simulink model "testharness"  (R2023a)
settings: Solver=ode4  StartTime=0.0  StopTime=30  FixedStep=sim.sample_time_s  RelTol=1e-3
undefined symbols (not defined in the file): rot_K_meas_IB_B_radDs, sfor_meas_B_mDs2, sim
libraries: simulink x5, lib_kinematics x2, matrix_library x1
settings Model: PauseTimes=16  Creator=FC_dev1  LastModifiedBy=FC_dev1

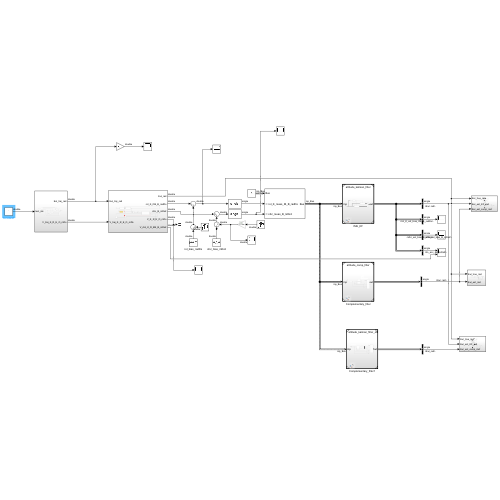
[thumbnail: Simulink's stored preview of the top-level diagram]
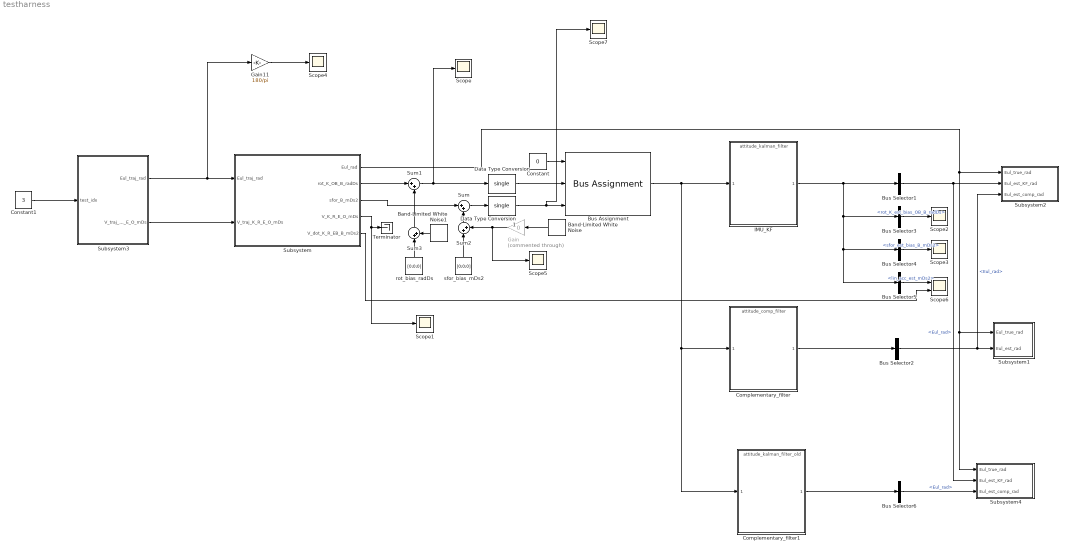
== system testharness ==
  Band-Limited White Noise : simulink/Sources/Band-Limited White Noise  Cov=meas_acc_var  Ts=0.1  seed=[1 2 3]
  Band-Limited White Noise1 : simulink/Sources/Band-Limited White Noise  Cov=rot_var  Ts=0.1  seed=[1 2 3]
  Bus Assignment : BusAssignment  AssignedSignals=rot_K_meas_IB_B_radDs,sfor_meas_B_mDs2
  Bus Selector1 : BusSelector  OutputSignals=Eul_rad
  Bus Selector2 : BusSelector  OutputSignals=Eul_rad
  Bus Selector3 : BusSelector  OutputSignals=rot_K_est_bias_OB_B_radDs
  Bus Selector4 : BusSelector  OutputSignals=sfor_est_bias_B_mDs2
  Bus Selector5 : BusSelector  OutputSignals=lin_acc_est_mDs2
  Bus Selector6 : BusSelector  OutputSignals=Eul_rad
  Complementary_filter : ModelReference  ModelNameDialog=attitude_comp_filter.slx  SimulationMode=Normal  ModelReferenceVersion=1.222
  Complementary_filter1 : ModelReference  ModelNameDialog=attitude_kalman_filter_old.slx  SimulationMode=Normal  ModelReferenceVersion=1.208
  Constant : Constant  Value=0  OutDataTypeStr=Bus: inp_Bus
  Constant1 : Constant  Value=3
  Data Type Conversion : DataTypeConversion  OutDataTypeStr=single  SaturateOnIntegerOverflow=off  RndMeth=Floor
  Data Type Conversion1 : DataTypeConversion  OutDataTypeStr=single  SaturateOnIntegerOverflow=off  RndMeth=Floor
  Gain : Gain  Commented=through  Gain=0
  Gain11 : Gain  Gain=180/pi
  IMU_KF : ModelReference  ModelNameDialog=attitude_kalman_filter.slx  SimulationMode=Normal  ModelReferenceVersion=1.336
  Scope{,1..5,7} (7 alike) : Scope
  Scope6 : Scope  NumInputPorts=2
  Subsystem : Subsystem
  Subsystem1 : Subsystem
  Subsystem2 : Subsystem
  Subsystem3 : Subsystem
  Subsystem4 : Subsystem
  Sum{,1..3} (4 alike) : Sum  Inputs=|++
  Terminator : Terminator
  rot_bias_radDs : Constant  Value=[0;0;0]  VectorParams1D=off
  sfor_bias_mDs2 : Constant  Value=[0;0;0]  VectorParams1D=off
  wires:
  Constant/1 -> Bus Assignment/1
  Bus Assignment/1 -> Complementary_filter1/1, Complementary_filter/1, IMU_KF/1
  Data Type Conversion/1 -> Bus Assignment/2
  Data Type Conversion1/1 -> Scope7/1, Bus Assignment/3
  Subsystem/1(Eul_rad) -> Subsystem4/1(Eul_true_rad), Subsystem1/1(Eul_true_rad), Subsystem2/1(Eul_true_rad)
  Subsystem/2(rot_K_OB_B_radDs) -> Sum1/1
  Subsystem/3(sfor_B_mDs2) -> Sum/1
  IMU_KF/1 -> Bus Selector3/1, Bus Selector5/1, Bus Selector4/1, Bus Selector1/1
  Bus Selector1/1 -> Subsystem4/2(Eul_est_KF_rad), Subsystem2/2(Eul_est_KF_rad)  "<Eul_rad>"
  Bus Selector3/1 -> Scope2/1  "<rot_K_est_bias_OB_B_radDs>"
  Bus Selector4/1 -> Scope3/1  "<sfor_est_bias_B_mDs2>"
  Gain11/1 -> Scope4/1
  Subsystem/4(V_K_R_E_O_mDs) -> Scope1/1, Terminator/1
  Sum/1 -> Data Type Conversion1/1
  Sum1/1 -> Data Type Conversion/1, Scope/1
  rot_bias_radDs/1 -> Sum3/1
  sfor_bias_mDs2/1 -> Sum2/1
  Complementary_filter/1 -> Bus Selector2/1
  Bus Selector2/1 -> Subsystem2/3(Eul_est_comp_rad), Subsystem1/2(Eul_est_rad)  "<Eul_rad>"
  Subsystem3/1(Eul_traj_rad) -> Gain11/1, Subsystem/1(Eul_traj_rad)
  Subsystem3/2(V_traj_K_R_E_O_mDs) -> Subsystem/2(V_traj_K_R_E_O_mDs)
  Constant1/1 -> Subsystem3/1(test_idx)
  Sum2/1 -> Sum/2
  Band-Limited White Noise/1 -> Gain/1
  Sum3/1 -> Sum1/2
  Band-Limited White Noise1/1 -> Sum3/2
  Complementary_filter1/1 -> Bus Selector6/1
  Bus Selector6/1 -> Subsystem4/3(Eul_est_comp_rad)  "<Eul_rad>"
  Bus Selector5/1 -> Scope6/1  "<lin_acc_est_mDs2>"
  Subsystem/5(V_dot_K_R_EB_B_mDs2) -> Scope6/2
  Gain/1 -> Scope5/1, Sum2/2

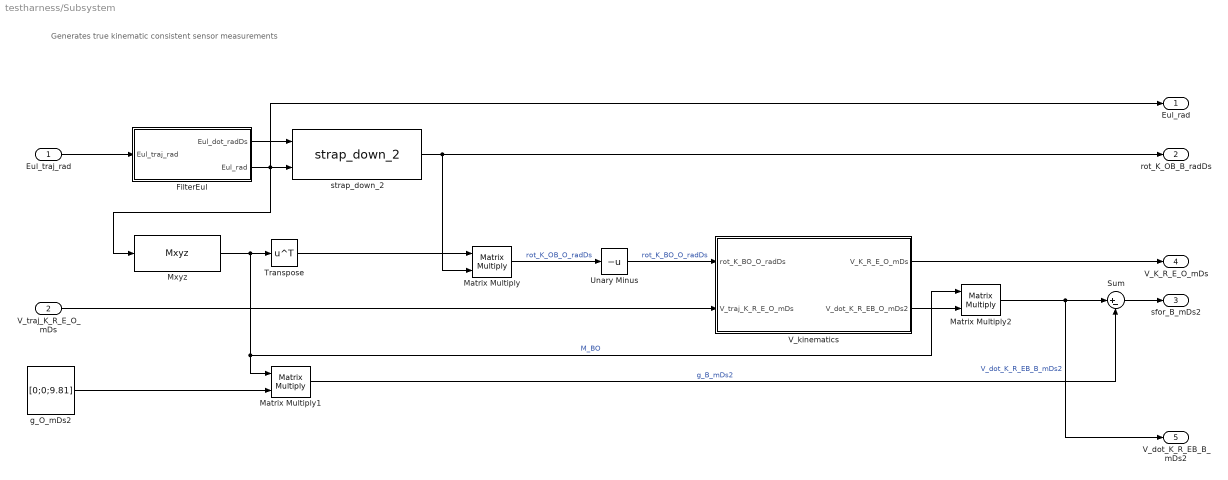
== system testharness/Subsystem ==
  note: Generates true kinematic consistent sensor measurements
  Eul_traj_rad : Inport
  V_traj_K_R_E_O_mDs : Inport  Port=2
  FilterEul : Subsystem
  Matrix Multiply : Product  Multiplication=Matrix(*)
  Matrix Multiply1 : Product  Multiplication=Matrix(*)
  Matrix Multiply2 : Product  Multiplication=Matrix(*)
  Mxyz : lib_kinematics/Mxyz  SystemSampleTime=-1  VariantActivationTime=update diagram  Latency=0  AutoFrameSizeCalculation=off
  Sum : Sum  Inputs=|+-
  Transpose : Math  Operator=transpose
  Unary Minus : UnaryMinus
  V_kinematics : Subsystem
  g_O_mDs2 : Constant  Value=[0;0;9.81]  VectorParams1D=off
  strap_down_2 : lib_kinematics/strap_down_2  SystemSampleTime=-1  VariantActivationTime=update diagram  Latency=0  AutoFrameSizeCalculation=off
  Eul_rad : Outport
  rot_K_OB_B_radDs : Outport  Port=2
  sfor_B_mDs2 : Outport  Port=3
  V_K_R_E_O_mDs : Outport  Port=4
  V_dot_K_R_EB_B_mDs2 : Outport  Port=5
  wires:
  Eul_traj_rad/1 -> FilterEul/1(Eul_traj_rad)
  V_traj_K_R_E_O_mDs/1 -> V_kinematics/2(V_traj_K_R_E_O_mDs)
  FilterEul/1(Eul_dot_radDs) -> strap_down_2/1
  FilterEul/2(Eul_rad) -> Mxyz/1, Eul_rad/1, strap_down_2/2
  Mxyz/1 -> Matrix Multiply2/1, Matrix Multiply1/1, Transpose/1  "M_BO"
  Transpose/1 -> Matrix Multiply/1
  strap_down_2/1 -> rot_K_OB_B_radDs/1, Matrix Multiply/2
  Matrix Multiply/1 -> Unary Minus/1  "rot_K_OB_O_radDs"
  Unary Minus/1 -> V_kinematics/1(rot_K_BO_O_radDs)  "rot_K_BO_O_radDs"
  g_O_mDs2/1 -> Matrix Multiply1/2
  Matrix Multiply1/1 -> Sum/2  "g_B_mDs2"
  Sum/1 -> sfor_B_mDs2/1
  V_kinematics/2(V_dot_K_R_EB_O_mDs2) -> Matrix Multiply2/2
  Matrix Multiply2/1 -> V_dot_K_R_EB_B_mDs2/1, Sum/1  "V_dot_K_R_EB_B_mDs2"
  V_kinematics/1(V_K_R_E_O_mDs) -> V_K_R_E_O_mDs/1

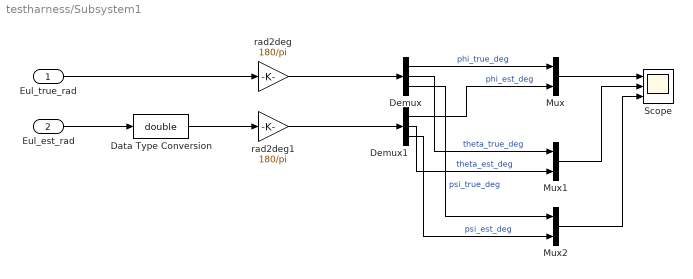
== system testharness/Subsystem1 ==
  Eul_true_rad : Inport
  Eul_est_rad : Inport  Port=2
  Data Type Conversion : DataTypeConversion  OutDataTypeStr=double  SaturateOnIntegerOverflow=off  RndMeth=Floor
  Demux : Demux  Outputs=3
  Demux1 : Demux  Outputs=3
  Mux : Mux  Inputs=2
  Mux1 : Mux  Inputs=2
  Mux2 : Mux  Inputs=2
  Scope : Scope  NumInputPorts=3
  rad2deg : Gain  Gain=180/pi  OutDataTypeStr=Inherit: Same as input
  rad2deg1 : Gain  Gain=180/pi  OutDataTypeStr=Inherit: Same as input
  wires:
  Eul_est_rad/1 -> Data Type Conversion/1
  Eul_true_rad/1 -> rad2deg/1
  rad2deg/1 -> Demux/1
  rad2deg1/1 -> Demux1/1
  Demux/1 -> Mux/1  "phi_true_deg"
  Demux1/1 -> Mux/2  "phi_est_deg"
  Demux/2 -> Mux1/1  "theta_true_deg"
  Demux1/2 -> Mux1/2  "theta_est_deg"
  Demux/3 -> Mux2/1  "psi_true_deg"
  Demux1/3 -> Mux2/2  "psi_est_deg"
  Mux/1 -> Scope/1
  Mux1/1 -> Scope/2
  Mux2/1 -> Scope/3
  Data Type Conversion/1 -> rad2deg1/1

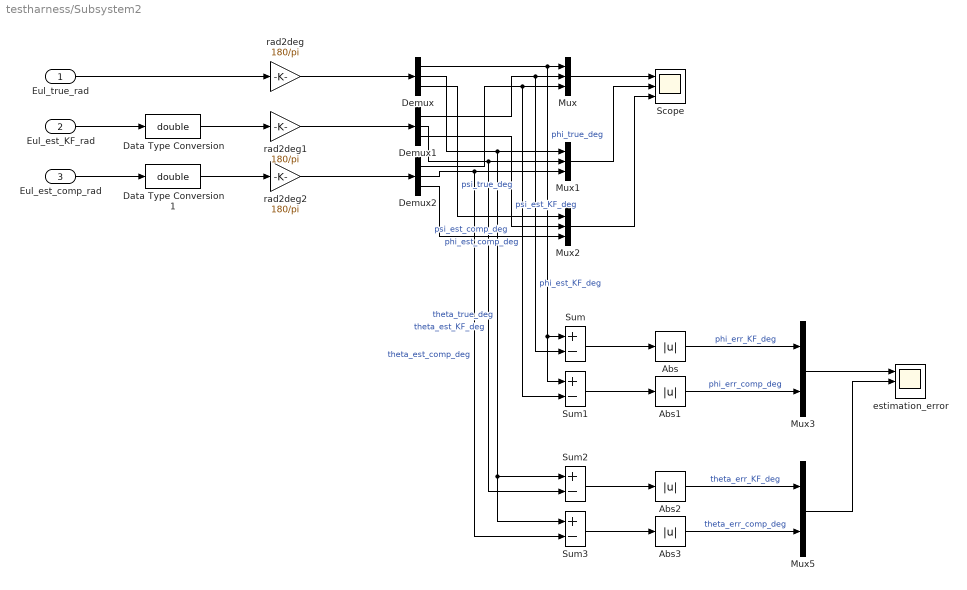
== system testharness/Subsystem2 ==
  Eul_true_rad : Inport
  Eul_est_KF_rad : Inport  Port=2
  Eul_est_comp_rad : Inport  Port=3
  Abs{,1..3} (4 alike) : Abs  SaturateOnIntegerOverflow=off
  Data Type Conversion : DataTypeConversion  OutDataTypeStr=double  SaturateOnIntegerOverflow=off  RndMeth=Floor
  Data Type Conversion1 : DataTypeConversion  OutDataTypeStr=double  SaturateOnIntegerOverflow=off  RndMeth=Floor
  Demux : Demux  Outputs=3
  Demux1 : Demux  Outputs=3
  Demux2 : Demux  Outputs=3
  Mux : Mux  Inputs=3
  Mux1 : Mux  Inputs=3
  Mux2 : Mux  Inputs=3
  Mux3 : Mux  Inputs=2
  Mux5 : Mux  Inputs=2
  Scope : Scope  NumInputPorts=3
  Sum{,1..3} (4 alike) : Sum  Inputs=+-
  estimation_error : Scope  NumInputPorts=3
  rad2deg : Gain  Gain=180/pi  OutDataTypeStr=Inherit: Same as input
  rad2deg1 : Gain  Gain=180/pi  OutDataTypeStr=Inherit: Same as input
  rad2deg2 : Gain  Gain=180/pi  OutDataTypeStr=Inherit: Same as input
  wires:
  Data Type Conversion/1 -> rad2deg1/1
  Mux2/1 -> Scope/3
  Mux1/1 -> Scope/2
  Mux/1 -> Scope/1
  Demux1/3 -> Mux2/2  "psi_est_KF_deg"
  Demux/3 -> Mux2/1  "psi_true_deg"
  Demux1/2 -> Sum2/2, Mux1/2  "theta_est_KF_deg"
  Demux/2 -> Sum3/1, Sum2/1, Mux1/1  "theta_true_deg"
  Demux1/1 -> Sum/2, Mux/2  "phi_est_KF_deg"
  Demux/1 -> Sum1/1, Sum/1, Mux/1  "phi_true_deg"
  rad2deg1/1 -> Demux1/1
  rad2deg/1 -> Demux/1
  Eul_true_rad/1 -> rad2deg/1
  Eul_est_KF_rad/1 -> Data Type Conversion/1
  Eul_est_comp_rad/1 -> Data Type Conversion1/1
  Data Type Conversion1/1 -> rad2deg2/1
  rad2deg2/1 -> Demux2/1
  Demux2/1 -> Sum1/2, Mux/3  "phi_est_comp_deg"
  Demux2/2 -> Mux1/3, Sum3/2  "theta_est_comp_deg"
  Demux2/3 -> Mux2/3  "psi_est_comp_deg"
  Sum/1 -> Abs/1
  Abs/1 -> Mux3/1  "phi_err_KF_deg"
  Sum1/1 -> Abs1/1
  Abs1/1 -> Mux3/2  "phi_err_comp_deg"
  Mux3/1 -> estimation_error/1
  Sum2/1 -> Abs2/1
  Sum3/1 -> Abs3/1
  Abs2/1 -> Mux5/1  "theta_err_KF_deg"
  Abs3/1 -> Mux5/2  "theta_err_comp_deg"
  Mux5/1 -> estimation_error/2

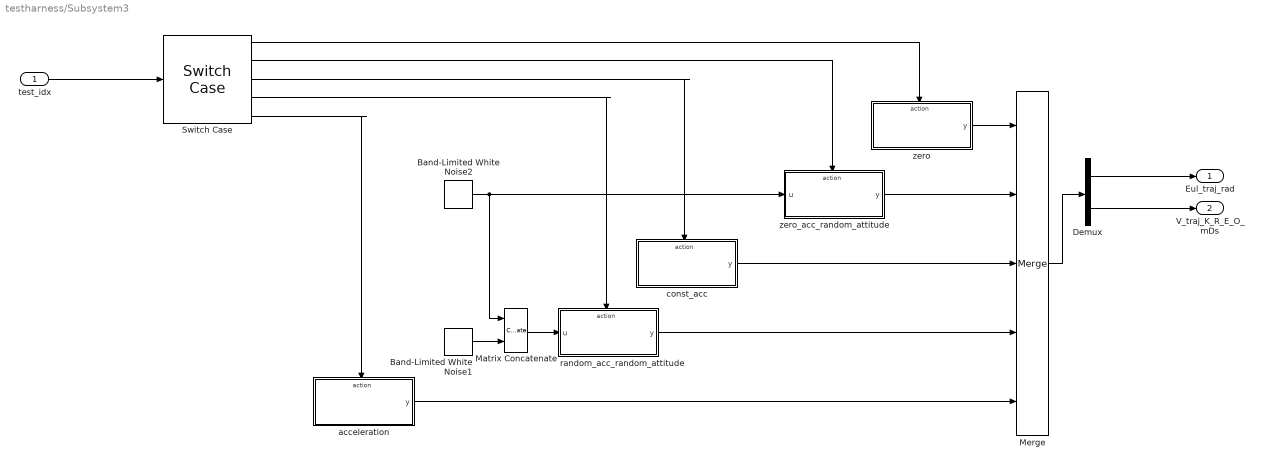
== system testharness/Subsystem3 ==
  test_idx : Inport
  Band-Limited White Noise1 : simulink/Sources/Band-Limited White Noise  Cov=[1 1 1]*5  Ts=sim.sample_time_s  seed=[23344 23345 23346]
  Band-Limited White Noise2 : simulink/Sources/Band-Limited White Noise  Cov=[0.01 0.01 0.01]  Ts=sim.sample_time_s  seed=[23341 23342 23343]
  Demux : Demux  Outputs=2
  Matrix Concatenate : Concatenate  Mode=Multidimensional array
  Merge : Merge  Inputs=5
  Switch Case : SwitchCase  CaseConditions={0,1,2,3,4}  ShowDefaultCase=off
  acceleration : Subsystem  TreatAsAtomicUnit=on
  const_acc : Subsystem  TreatAsAtomicUnit=on
  random_acc_random_attitude : Subsystem  TreatAsAtomicUnit=on
  zero : Subsystem  TreatAsAtomicUnit=on
  zero_acc_random_attitude : Subsystem  TreatAsAtomicUnit=on
  Eul_traj_rad : Outport
  V_traj_K_R_E_O_mDs : Outport  Port=2
  wires:
  test_idx/1 -> Switch Case/1
  Switch Case/3 -> const_acc/Action
  Switch Case/2 -> zero_acc_random_attitude/Action
  Switch Case/1 -> zero/Action
  zero/1(y) -> Merge/1
  zero_acc_random_attitude/1(y) -> Merge/2
  const_acc/1(y) -> Merge/3
  Merge/1 -> Demux/1
  Demux/1 -> Eul_traj_rad/1
  Demux/2 -> V_traj_K_R_E_O_mDs/1
  Band-Limited White Noise2/1 -> Matrix Concatenate/1, zero_acc_random_attitude/1(u)
  random_acc_random_attitude/1(y) -> Merge/4
  Switch Case/4 -> random_acc_random_attitude/Action
  Band-Limited White Noise1/1 -> Matrix Concatenate/2
  Matrix Concatenate/1 -> random_acc_random_attitude/1(u)
  acceleration/1(y) -> Merge/5
  Switch Case/5 -> acceleration/Action

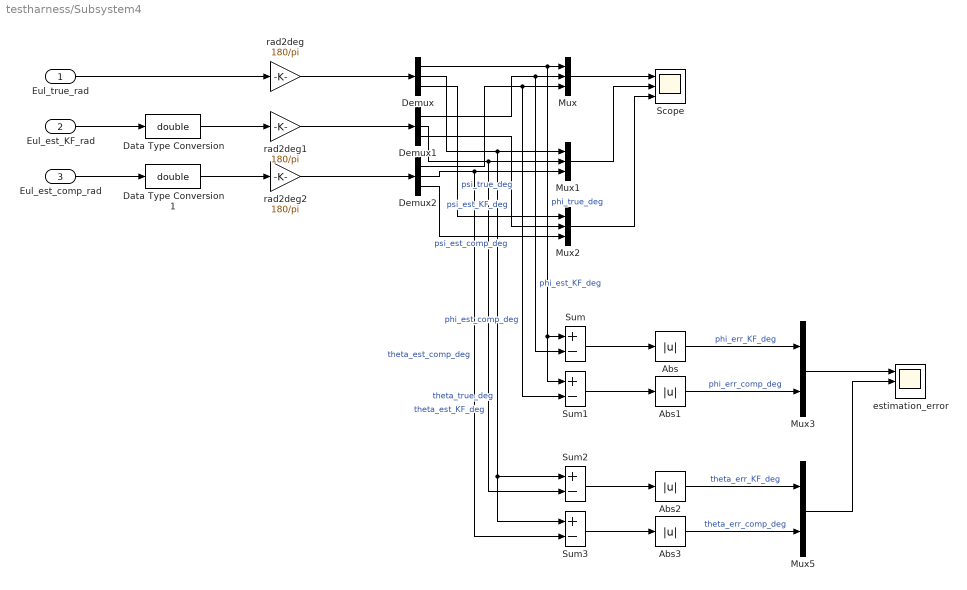
== system testharness/Subsystem4 ==
  Eul_true_rad : Inport
  Eul_est_KF_rad : Inport  Port=2
  Eul_est_comp_rad : Inport  Port=3
  Abs{,1..3} (4 alike) : Abs  SaturateOnIntegerOverflow=off
  Data Type Conversion : DataTypeConversion  OutDataTypeStr=double  SaturateOnIntegerOverflow=off  RndMeth=Floor
  Data Type Conversion1 : DataTypeConversion  OutDataTypeStr=double  SaturateOnIntegerOverflow=off  RndMeth=Floor
  Demux : Demux  Outputs=3
  Demux1 : Demux  Outputs=3
  Demux2 : Demux  Outputs=3
  Mux : Mux  Inputs=3
  Mux1 : Mux  Inputs=3
  Mux2 : Mux  Inputs=3
  Mux3 : Mux  Inputs=2
  Mux5 : Mux  Inputs=2
  Scope : Scope  NumInputPorts=3
  Sum{,1..3} (4 alike) : Sum  Inputs=+-
  estimation_error : Scope  NumInputPorts=3
  rad2deg : Gain  Gain=180/pi  OutDataTypeStr=Inherit: Same as input
  rad2deg1 : Gain  Gain=180/pi  OutDataTypeStr=Inherit: Same as input
  rad2deg2 : Gain  Gain=180/pi  OutDataTypeStr=Inherit: Same as input
  wires:
  Mux5/1 -> estimation_error/2
  Abs3/1 -> Mux5/2  "theta_err_comp_deg"
  Abs2/1 -> Mux5/1  "theta_err_KF_deg"
  Sum3/1 -> Abs3/1
  Sum2/1 -> Abs2/1
  Mux3/1 -> estimation_error/1
  Abs1/1 -> Mux3/2  "phi_err_comp_deg"
  Sum1/1 -> Abs1/1
  Abs/1 -> Mux3/1  "phi_err_KF_deg"
  Sum/1 -> Abs/1
  Demux2/3 -> Mux2/3  "psi_est_comp_deg"
  Demux2/2 -> Sum3/2, Mux1/3  "theta_est_comp_deg"
  Demux2/1 -> Mux/3, Sum1/2  "phi_est_comp_deg"
  rad2deg2/1 -> Demux2/1
  Data Type Conversion1/1 -> rad2deg2/1
  Eul_est_comp_rad/1 -> Data Type Conversion1/1
  Eul_est_KF_rad/1 -> Data Type Conversion/1
  Eul_true_rad/1 -> rad2deg/1
  rad2deg/1 -> Demux/1
  rad2deg1/1 -> Demux1/1
  Demux/1 -> Mux/1, Sum/1, Sum1/1  "phi_true_deg"
  Demux1/1 -> Mux/2, Sum/2  "phi_est_KF_deg"
  Demux/2 -> Mux1/1, Sum2/1, Sum3/1  "theta_true_deg"
  Demux1/2 -> Mux1/2, Sum2/2  "theta_est_KF_deg"
  Demux/3 -> Mux2/1  "psi_true_deg"
  Demux1/3 -> Mux2/2  "psi_est_KF_deg"
  Mux/1 -> Scope/1
  Mux1/1 -> Scope/2
  Mux2/1 -> Scope/3
  Data Type Conversion/1 -> rad2deg1/1

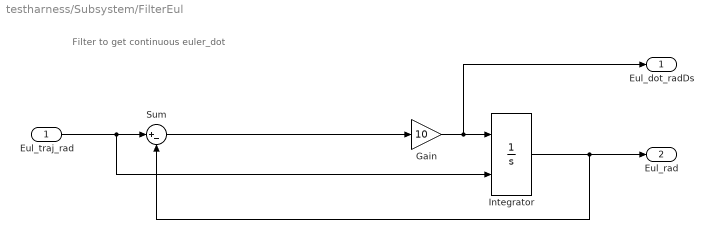
== system testharness/Subsystem/FilterEul ==
  note: Filter to get continuous euler_dot
  Eul_traj_rad : Inport
  Gain : Gain  Gain=10
  Integrator : Integrator  InitialConditionSource=external  WrappedStateUpperValue=[pi; pi/2; 2*pi]  WrappedStateLowerValue=[-pi; -pi/2; 0]
  Sum : Sum  Inputs=|+-
  Eul_dot_radDs : Outport
  Eul_rad : Outport  Port=2
  wires:
  Eul_traj_rad/1 -> Integrator/2, Sum/1
  Gain/1 -> Eul_dot_radDs/1, Integrator/1
  Integrator/1 -> Eul_rad/1, Sum/2
  Sum/1 -> Gain/1

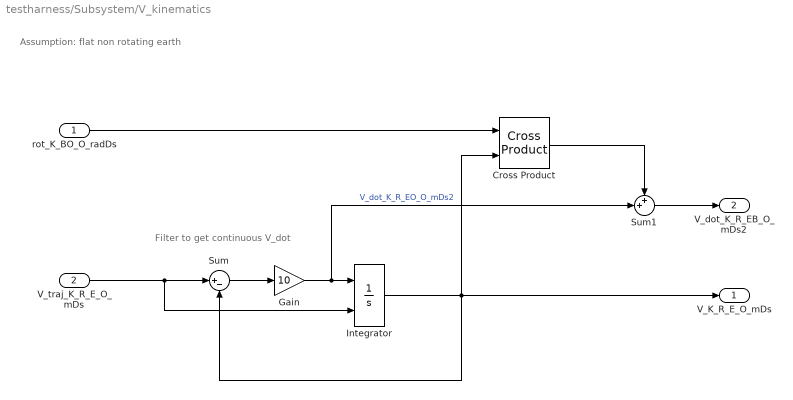
== system testharness/Subsystem/V_kinematics ==
  note: Assumption: flat non rotating earth
  note: Filter to get continuous V_dot
  rot_K_BO_O_radDs : Inport
  V_traj_K_R_E_O_mDs : Inport  Port=2
  Cross Product : matrix_library/Cross Product
  Gain : Gain  Gain=10
  Integrator : Integrator  InitialConditionSource=external
  Sum : Sum  Inputs=|+-
  Sum1 : Sum  Inputs=++|
  V_K_R_E_O_mDs : Outport
  V_dot_K_R_EB_O_mDs2 : Outport  Port=2
  wires:
  V_traj_K_R_E_O_mDs/1 -> Sum/1, Integrator/2
  Sum/1 -> Gain/1
  Gain/1 -> Sum1/2, Integrator/1  "V_dot_K_R_EO_O_mDs2"
  Integrator/1 -> Cross Product/2, Sum/2, V_K_R_E_O_mDs/1
  rot_K_BO_O_radDs/1 -> Cross Product/1
  Sum1/1 -> V_dot_K_R_EB_O_mDs2/1
  Cross Product/1 -> Sum1/1

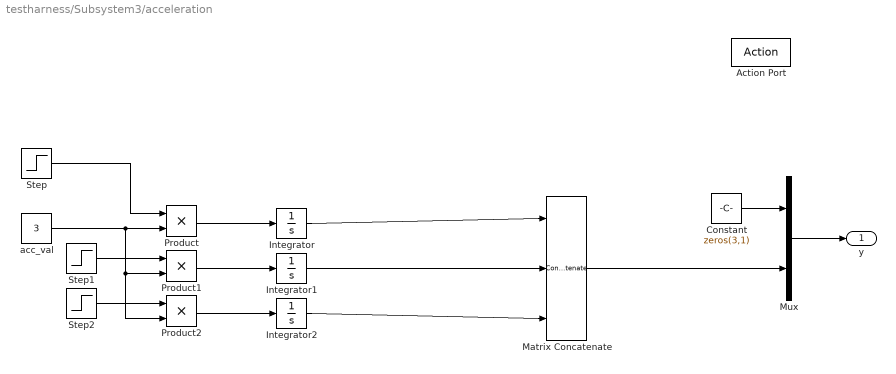
== system testharness/Subsystem3/acceleration ==
  Action Port : ActionPort  ActionPortLabel=case [ 4 ]:
  Constant : Constant  Value=zeros(3,1)  VectorParams1D=off
  Integrator : Integrator  LimitOutput=on  UpperSaturationLimit=20  LowerSaturationLimit=-20
  Integrator1 : Integrator  LimitOutput=on  UpperSaturationLimit=20  LowerSaturationLimit=-20
  Integrator2 : Integrator  LimitOutput=on  UpperSaturationLimit=20  LowerSaturationLimit=-20
  Matrix Concatenate : Concatenate  NumInputs=3  Mode=Multidimensional array
  Mux : Mux  Inputs=2
  Product : Product
  Product1 : Product
  Product2 : Product
  Step : Step  SampleTime=0
  Step1 : Step  Time=10  SampleTime=0
  Step2 : Step  Time=20  SampleTime=0
  acc_val : Constant  Value=3
  y : Outport
  wires:
  Matrix Concatenate/1 -> Mux/2
  Mux/1 -> y/1
  Constant/1 -> Mux/1
  acc_val/1 -> Product2/2, Product1/2, Product/2
  Step/1 -> Product/1
  Product/1 -> Integrator/1
  Integrator/1 -> Matrix Concatenate/1
  Integrator1/1 -> Matrix Concatenate/2
  Integrator2/1 -> Matrix Concatenate/3
  Product1/1 -> Integrator1/1
  Product2/1 -> Integrator2/1
  Step1/1 -> Product1/1
  Step2/1 -> Product2/1

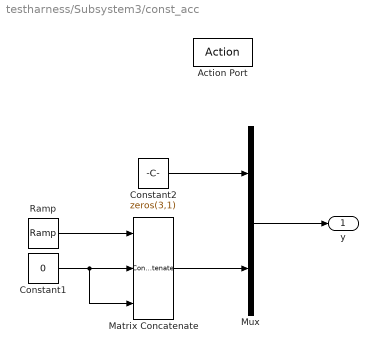
== system testharness/Subsystem3/const_acc ==
  Action Port : ActionPort  ActionPortLabel=case [ 2 ]:
  Constant1 : Constant  Value=0  VectorParams1D=off
  Constant2 : Constant  Value=zeros(3,1)  VectorParams1D=off
  Matrix Concatenate : Concatenate  NumInputs=3  Mode=Multidimensional array
  Mux : Mux  Inputs=2
  Ramp : simulink/Sources/Ramp  slope=1  start=1  InitialOutput=0
  y : Outport
  wires:
  Mux/1 -> y/1
  Constant2/1 -> Mux/1
  Matrix Concatenate/1 -> Mux/2
  Ramp/1 -> Matrix Concatenate/1
  Constant1/1 -> Matrix Concatenate/3, Matrix Concatenate/2

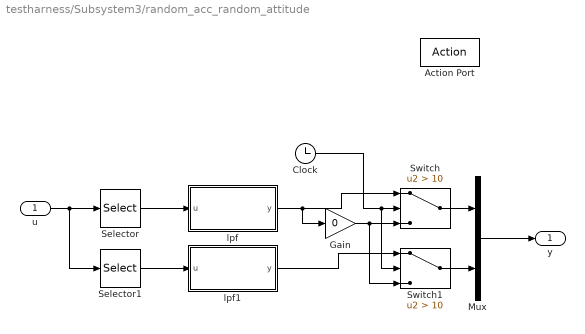
== system testharness/Subsystem3/random_acc_random_attitude ==
  u : Inport
  Action Port : ActionPort  ActionPortLabel=case [ 3 ]:
  Clock : Clock
  Gain : Gain  Gain=0
  Mux : Mux  Inputs=2
  Selector : Selector  NumberOfDimensions=2  InputPortWidth=3  IndexOptions=Index vector (dialog),Index vector (dialog)  Indices=1:3,1  OutputSizes=1,1
  Selector1 : Selector  NumberOfDimensions=2  InputPortWidth=3  IndexOptions=Index vector (dialog),Index vector (dialog)  Indices=4:6,1  OutputSizes=1,1
  Switch : Switch  Criteria=u2 > Threshold  Threshold=10  SaturateOnIntegerOverflow=off  InputSameDT=off
  Switch1 : Switch  Criteria=u2 > Threshold  Threshold=10  SaturateOnIntegerOverflow=off  InputSameDT=off
  lpf : Subsystem
  lpf1 : Subsystem
  y : Outport
  wires:
  Mux/1 -> y/1
  u/1 -> Selector1/1, Selector/1
  lpf/1(y) -> Switch/1, Gain/1
  Selector/1 -> lpf/1(u)
  Selector1/1 -> lpf1/1(u)
  lpf1/1(y) -> Switch1/1
  Clock/1 -> Switch1/2, Switch/2
  Switch/1 -> Mux/1
  Gain/1 -> Switch1/3, Switch/3
  Switch1/1 -> Mux/2

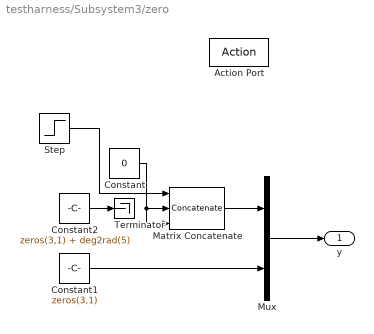
== system testharness/Subsystem3/zero ==
  Action Port : ActionPort  ActionPortLabel=case [ 0 ]:
  Constant : Constant  Value=0
  Constant1 : Constant  Value=zeros(3,1)  VectorParams1D=off
  Constant2 : Constant  Value=zeros(3,1) + deg2rad(5)  VectorParams1D=off
  Matrix Concatenate : Concatenate  NumInputs=3  Mode=Multidimensional array
  Mux : Mux  Inputs=2
  Step : Step  Time=2  After=deg2rad(180)  SampleTime=0
  Terminator : Terminator
  y : Outport
  wires:
  Constant1/1 -> Mux/2
  Mux/1 -> y/1
  Matrix Concatenate/1 -> Mux/1
  Constant2/1 -> Terminator/1
  Step/1 -> Matrix Concatenate/1
  Constant/1 -> Matrix Concatenate/2, Matrix Concatenate/3

== system testharness/Subsystem3/zero_acc_random_attitude ==
  u : Inport
  Action Port : ActionPort  ActionPortLabel=case [ 1 ]:
  Constant1 : Constant  Value=zeros(3,1)  VectorParams1D=off
  Mux : Mux  Inputs=2
  lpf : Subsystem
  y : Outport
  wires:
  lpf/1(y) -> Mux/1
  Constant1/1 -> Mux/2
  u/1 -> lpf/1(u)
  Mux/1 -> y/1

== system testharness/Subsystem3/random_acc_random_attitude/lpf ==
  u : Inport
  Gain : Gain  Gain=0.5
  Integrator : Integrator
  Sum : Sum  Inputs=|+-
  y : Outport
  wires:
  Integrator/1 -> y/1, Sum/2
  Gain/1 -> Integrator/1
  Sum/1 -> Gain/1
  u/1 -> Sum/1

== system testharness/Subsystem3/random_acc_random_attitude/lpf1 ==
  u : Inport
  Gain : Gain  Gain=0.01
  Integrator : Integrator
  Sum : Sum  Inputs=|+-
  y : Outport
  wires:
  u/1 -> Sum/1
  Sum/1 -> Gain/1
  Gain/1 -> Integrator/1
  Integrator/1 -> Sum/2, y/1

== system testharness/Subsystem3/zero_acc_random_attitude/lpf ==
  u : Inport
  Gain : Gain  Gain=0.5
  Integrator : Integrator
  Sum : Sum  Inputs=|+-
  y : Outport
  wires:
  u/1 -> Sum/1
  Sum/1 -> Gain/1
  Gain/1 -> Integrator/1
  Integrator/1 -> Sum/2, y/1
